simulink model "controlador_malha_aberta_21_a"  (R2021a)
settings: Solver=VariableStepAuto  StartTime=0.0  StopTime=2  RelTol=1e-3
undefined symbols (not defined in the file or in its folder): K_barra, Ka, Kp, Kt, tau
settings Model: Creator=carol  LastModifiedBy=Guilherme

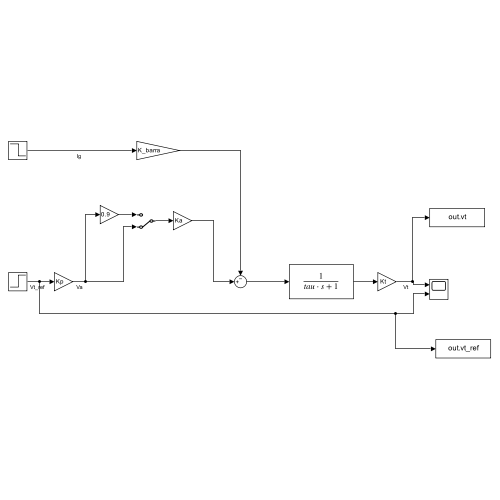
[thumbnail: Simulink's stored preview of the top-level diagram]
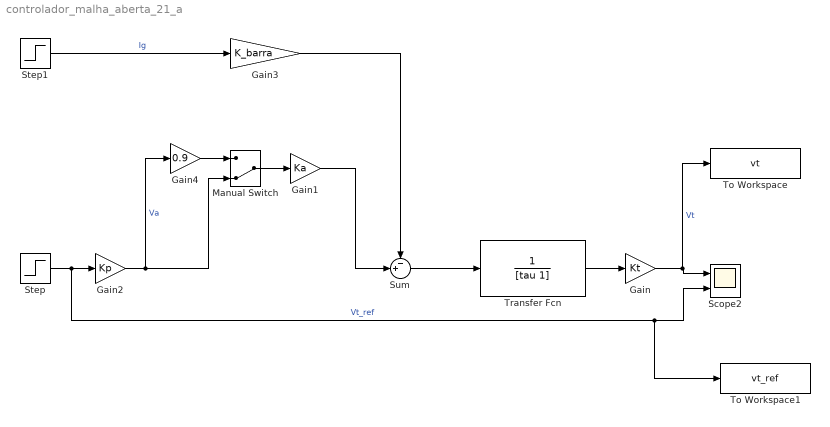
== system controlador_malha_aberta_21_a ==
  Gain : Gain  Gain=Kt
  Gain1 : Gain  Gain=Ka
  Gain2 : Gain  Gain=Kp
  Gain3 : Gain  Gain=K_barra
  Gain4 : Gain  Gain=0.9
  Manual Switch : ManualSwitch  CurrentSetting=0
  Scope2 : Scope  NumInputPorts=2
  Step : Step  Time=0  After=10  SampleTime=0
  Step1 : Step  Time=0  Before=0.450  After=0  SampleTime=0
  Sum : Sum  Inputs=-+|
  To Workspace : ToWorkspace  VariableName=vt  SaveFormat=Timeseries  SampleTime=-1
  To Workspace1 : ToWorkspace  VariableName=vt_ref  SaveFormat=Timeseries  SampleTime=-1
  Transfer Fcn : TransferFcn  Denominator=[tau 1]
  wires:
  Transfer Fcn/1 -> Gain/1
  Gain/1 -> To Workspace/1, Scope2/1  "Vt"
  Sum/1 -> Transfer Fcn/1
  Gain1/1 -> Sum/2
  Step/1 -> Gain2/1, To Workspace1/1, Scope2/2  "Vt_ref"
  Step1/1 -> Gain3/1  "Ig"
  Gain3/1 -> Sum/1
  Manual Switch/1 -> Gain1/1
  Gain2/1 -> Gain4/1, Manual Switch/2  "Va"
  Gain4/1 -> Manual Switch/1
